simulink model "Longitudinal_Example_V5"  (R2016a)
settings: Solver=ode45  StartTime=0.0  StopTime=40  RelTol=1e-3
InitFcn:
  | Longitudinal_Example_V2
  | Lateral_Example_V2
  | Pre_3D_Visualisation
values from neighbouring files (symbols this model uses):
  A_Lat = [Yv,               Yp,               -(u0 - Yr),              g;          Lv,               Lp,               Lr,                      0;          Nv,               Np,               Nr,                      0;          0,                1,                0,                       0]    [Lateral_Example_V2.m]
  A_Lon = [Xu,               Xw,               0,              -g;      Zu,               Zw,               u0,              0;      Mu + (Mw_dot*Zu), Mw + (Mw_dot*Zw), Mq + Mw_dot*u0,  0;      0,                0,                1,               0]    [Longitudinal_Example_V2.m]
  B_Lat = zeros(4,2)    [Lateral_Example_V2.m]
  B_Lon = zeros(4,2)    [Longitudinal_Example_V2.m]
  C_Lat = eye(4)    [Lateral_Example_V2.m]
  C_Lon = eye(4)    [Longitudinal_Example_V2.m]
  D_Lat = zeros(4,2)    [Lateral_Example_V2.m]
  D_Lon = zeros(4,2)    [Longitudinal_Example_V2.m]
  initial = [u0; 0; 0; 0; 0; 0; 0; 0]    [Longitudinal_Example_V2.m]
  V = V./(scale_factor*correction)    [Pre_3D_Visualisation.m]
  x0_Lat = [0 0 0 0*(pi/180)]    [Lateral_Example_V2.m]
  x0_Lon = [8.2 0 0 0]    [Longitudinal_Example_V2.m]
undefined symbols (not defined in the file or in its folder): F
libraries: simulink x2, realtime_pacer_lib x1
settings Model: Creator=p-narayan  LastModifiedBy=sjm2-skilling
settings DataIOCC: LimitDataPoints=on  SaveFormat=Array
settings DebuggingCC: SolverPrmCheckMsg=warning  AllowSymbolicDim=off
settings HardwareCC: ProdBitPerPointer=32  ProdLargestAtomicFloat=None  ProdIntDivRoundTo=Undefined  ProdEndianess=Unspecified  ProdWordSize=32  ProdHWDeviceType=32-bit Generic
settings ModelReferenceCC: PropagateSignalLabelsOutOfModel=off
settings ConfigComp: CovModelRefEnable=Off  CovSFcnEnable=off

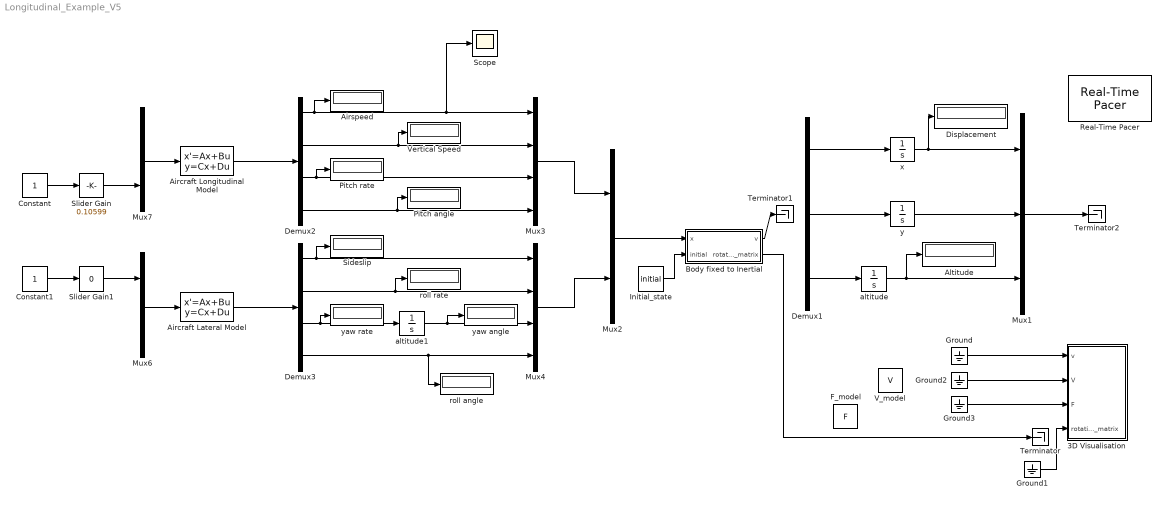
== system Longitudinal_Example_V5 ==
  3D Visualisation : MATLAB Function  TreatAsAtomicUnit=on
  Aircraft Lateral Model : StateSpace  A=A_Lat  B=B_Lat  C=C_Lat  D=D_Lat  X0=x0_Lat
  Aircraft Longitudinal Model : StateSpace  A=A_Lon  B=B_Lon  C=C_Lon  D=D_Lon  X0=x0_Lon
  Airspeed : Display
  Altitude : Display
  Body fixed to Inertial : MATLAB Function  TreatAsAtomicUnit=on
  Constant : Constant
  Constant1 : Constant
  Demux1 : Demux  Outputs=3
  Demux2 : Demux
  Demux3 : Demux
  Displacement : Display
  F_model : Constant  Value=F
  Ground{,1..3} (4 alike) : Ground
  Initial_state : Constant  Value=initial  SampleTime=0.1
  Mux1 : Mux  Inputs=3
  Mux2 : Mux  Inputs=2
  Mux3 : Mux
  Mux4 : Mux
  Mux6 : Mux  Inputs=2
  Mux7 : Mux  Inputs=2
  Pitch angle : Display
  Pitch rate : Display
  Real-Time Pacer : realtime_pacer_lib/Real-Time Pacer  simTimePerRealTime=5
  Scope : Scope
  Sideslip : Display
  Slider Gain : simulink/Math Operations/Slider Gain  low=-1  gain=0.10599  high=1
  Slider Gain1 : simulink/Math Operations/Slider Gain  low=-1  gain=0  high=1
  Terminator : Terminator
  Terminator1 : Terminator
  Terminator2 : Terminator
  "V_model " : Constant  Value=V
  Vertical Speed : Display
  altitude : Integrator  InitialCondition=500  ContinuousStateAttributes='altitude'
  altitude1 : Integrator  ContinuousStateAttributes='altitude'
  roll angle : Display
  roll rate : Display
  x : Integrator
  y : Integrator
  yaw angle : Display
  yaw rate : Display
  wires:
  Demux1/1 -> x/1
  Demux1/2 -> y/1
  Demux1/3 -> altitude/1
  altitude/1 -> Altitude/1, Mux1/3
  y/1 -> Mux1/2
  Initial_state/1 -> Body fixed to Inertial/2(initial)
  x/1 -> Displacement/1, Mux1/1
  Mux2/1 -> Body fixed to Inertial/1(x)
  Aircraft Longitudinal Model/1 -> Demux2/1
  Aircraft Lateral Model/1 -> Demux3/1
  Demux2/1 -> Scope/1, Mux3/1, Airspeed/1
  Demux2/2 -> Vertical Speed/1, Mux3/2
  Demux2/3 -> Pitch rate/1, Mux3/3
  Demux2/4 -> Pitch angle/1, Mux3/4
  Demux3/1 -> Sideslip/1, Mux4/1
  Demux3/2 -> roll rate/1, Mux4/2
  Demux3/3 -> yaw rate/1, altitude1/1
  Demux3/4 -> roll angle/1, Mux4/4
  altitude1/1 -> yaw angle/1, Mux4/3
  Mux3/1 -> Mux2/1
  Mux4/1 -> Mux2/2
  Mux7/1 -> Aircraft Longitudinal Model/1
  Mux6/1 -> Aircraft Lateral Model/1
  Constant/1 -> Slider Gain/1
  Slider Gain/1 -> Mux7/2
  Constant1/1 -> Slider Gain1/1
  Slider Gain1/1 -> Mux6/1
  Body fixed to Inertial/2(rotation_matrix) -> Terminator/1
  Body fixed to Inertial/1(v) -> Terminator1/1
  Mux1/1 -> Terminator2/1
  Ground/1 -> 3D Visualisation/1(v)
  Ground1/1 -> 3D Visualisation/4(rotation_matrix)
  Ground2/1 -> 3D Visualisation/2(V)
  Ground3/1 -> 3D Visualisation/3(F)

== matlab function Longitudinal_Example_V5/3D Visualisation ==
  data: v input; V input; F input; rotation_matrix input
function fcn(v, V, F, rotation_matrix)
% function fcn(v, V, F, rotation_matrix)
% %#codegen
% 
% % opengl hardware
% coder.extrinsic('patch')
% coder.extrinsic('delete')
% coder.extrinsic('exist')
% 
% cla
% 
% % Frame = struct('cdata',zeros(420,560,3));
% 
% %
% % x = u(1);
% % z = u(2);
% % q = u(3);
% % pitch = u(4);
% 
% x = v(1);
% y = v(2);
% z = v(3);
% % % pitch = v(4);
% % % roll = 0;
% % % yaw = 0;
% % % scale_factor = 1;
% % % step = 0.1;
% % selector
% 
% % coder.extrinsic('set_param');
% % coder.extrinsic('trajectory3');
% % coder.extrinsic('delete');
% 
% % =========================================================================
% 
% % trajectory3(x,0,z,pitch,0,0,0.2,0.1,'helicopter')
% 
% % trajectory3(x,y,z,pitch,roll,yaw,scale_factor,step,selector,varargin);
% 
% % mov=nargout;
% 
% %  strcmp(selector,'helicopter')
% %     load helicopter;
% % % V_AC=[-V(:,2) V(:,1) V(:,3)];
% % % V_AC(:,1)=V_AC(:,1)-round(sum(V_AC(:,1))/size(V_AC,1));
% % % V_AC(:,2)=V_AC(:,2)-round(sum(V_AC(:,2))/size(V_AC,1));
% % % V_AC(:,3)=V_AC(:,3)-round(sum(V_AC(:,3))/size(V_AC,1));
% % % 
% % % correction=max(abs(V_AC(:,1)));
% % % V_AC=V_AC./(scale_factor*correction);
% % ii=length(x);
% % resto=mod(ii,step);
% 
% %%%%%%%%%%%%%%%needed for the transformation%%%%%%%%%%%%%%%
% 
% % y=y;
% % z=z;
% % pitch=pitch;
% % roll=roll;
% % % yaw=-yaw;
% 
% %%%%%%%%%%%%%%%%%%%%%%%%%%%%%%%%%%%%%%%%%%%%%%%%%%%%%%%%%%%%
% 
% % % frame = 0;
% % for i=1:step:(ii-resto)
% %     if mov | (i == 1)
% %         clf;
% %         plot3(x,y,z);
% %         grid on;
% %         hold on;
% %         light;
% %     end
% 
% % % theta=pitch;
% % % phi=-roll;
% % % psi=yaw;
% 
% 
% Vnew=V*rotation_matrix;
% % Vnew=V;
% rif=[x y z];
% X0=repmat(rif,size(Vnew,1),1);
% Vnew=Vnew+X0;
% 
% p = patch('faces', F, 'vertices' ,Vnew);
% set(p, 'facec', [0 0 1]);
% set(p, 'EdgeColor','none');
% 
% % output = getframe(1);
% % outputfile =  
% % imwrite(img, 'outputfile.jpg');
% % Frame = [1 1];
% 
% 
% 
% 
% 
% % if mov | (i == 1)
% %     view(theView);
% %     axis equal;
% % end
% 
% % if mov
% %     if i == 1
% %         ax = axis;
% %     else
% %         axis(ax);
% %     end
% %     lighting phong
% %     frame = frame + 1;
% %     M(frame) = getframe;
% % end
% 
% % end
% 
% % hold on;
% % plot3(x,y,z);
% 
% % view(theView);
% % daspect([1 1 1]) ;
% % xlabel('X');
% % ylabel('Y');
% % zlabel('Z');
% 
% % cd (cur_dir);
% 
% % =========================================================================
% 
% 
% % axis([-10 10 -1 1 450 550])

== matlab function Longitudinal_Example_V5/Body fixed to Inertial ==
  data: x input; v output; initial input; rotation_matrix output
function [v, rotation_matrix] = fcn(x, initial)
%#codegen

% xdot = Ax + Bu
% where x = [Delta_u, Delta_w, Delta_q, Delta_theta]
% and y = [x_dot, y_dot, z_dot, Delta_theta]     % aircraft speed in
% inertial axis and pitch angle

theta = x(4)+initial(4);
psi = x(7)+initial(7);
phi = x(8)+initial(8);
    
u_b = x(1)+initial(1);
v_b = x(5)+initial(5);
w_b = x(2)+initial(2);

uvw_b = [u_b; v_b; w_b];

q0 = cos(phi/2)*cos(theta/2)*cos(psi/2)+sin(phi/2)*sin(theta/2)*sin(psi/2);
q1 = sin(phi/2)*cos(theta/2)*cos(psi/2)-cos(phi/2)*sin(theta/2)*sin(psi/2);
q2 = cos(phi/2)*sin(theta/2)*cos(psi/2)+sin(phi/2)*cos(theta/2)*sin(psi/2);
q3 = cos(phi/2)*sin(theta/2)*sin(psi/2)-sin(phi/2)*sin(theta/2)*cos(psi/2);

r11 = q0^2+q1^2-q2^2-q3^2;
r12 = 2*(q1*q2-q0*q3);
r13 = 2*(q0*q2+q1*q3);

r21 = 2*(q1*q2+q0*q3);
r22 = q0^2-q1^2+q2^2-q3^2;
r23 = 2*(q2*q3-q0*q1);

r31 = 2*(q1*q3-q0*q2);
r32 = 2*(q0*q1-q2*q3);
r33 = q0^2-q1^2-q2^2+q3^2;

rotation_matrix = [r11, r12, r13;...
                   r21, r22, r23;...
                   r31, r32, r33];

v = rotation_matrix*uvw_b;

% v = [v_i(1), v_i(2), v_i(3)];
